simulink model "test"  (R2024b)
settings: Solver=VariableStepAuto  StartTime=0.0  StopTime=10.0  RelTol=1e-3
libraries: cstblocks x3
settings Model: Creator=1163390615  LastModifiedBy=1163390615

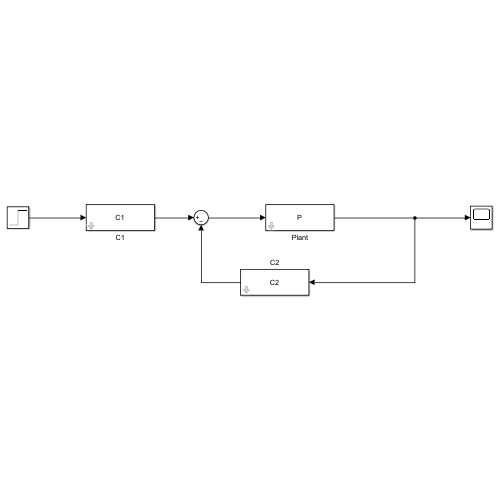
[thumbnail: Simulink's stored preview of the top-level diagram]
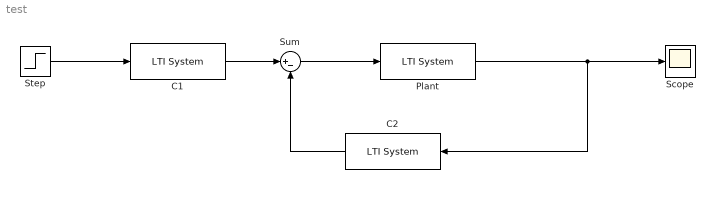
== system test ==
  C1 : cstblocks/LTI System  sys=C1  IC=[]  PadeOrder=0
  C2 : cstblocks/LTI System  sys=C2  IC=[]  PadeOrder=0
  Plant : cstblocks/LTI System  sys=P  IC=[]  PadeOrder=0
  Scope : Scope
  Step : Step  SampleTime=0
  Sum : Sum  Inputs=|+-
  wires:
  Step/1 -> C1/1
  Plant/1 -> C2/1, Scope/1
  C1/1 -> Sum/1
  C2/1 -> Sum/2
  Sum/1 -> Plant/1
